simulink model "HPUn_QntBalInjLim"  (R2016b)
settings: configuration reference "CodeGenConfigSet" (kept outside this file)
values from neighbouring files (symbols this model uses):
  HPUn_facPresDvtFlt_C = Calibration.Parameter    [init_HPUn_QntBalInjLim.m]    (also in init_HPUn_QntBalInjLim_SIL.m = Simulink.Parameter)
  HPUn_numInjMin_C = Calibration.Parameter    [init_HPUn_QntBalInjLim.m]    (also in init_HPUn_QntBalInjLim_SIL.m = Simulink.Parameter)
  HPUn_pRailDvtOk_C = Calibration.Parameter    [init_HPUn_QntBalInjLim.m]    (also in init_HPUn_QntBalInjLim_SIL.m = Simulink.Parameter)
  HPUn_tiQntBalDel_C = Calibration.Parameter    [init_HPUn_QntBalInjLim.m]    (also in init_HPUn_QntBalInjLim_SIL.m = Simulink.Parameter)
  InjCrv_numInjMaxSys_C = Calibration.Parameter    [init_HPUn_QntBalInjLim.m]    (also in init_HPUn_QntBalInjLim_SIL.m = Simulink.Parameter)
undefined symbols (not defined in the file or in its folder): HPUn_QntBalInjLim_DT
libraries: CXLib x1
settings Model: Creator=lenovo  LastModifiedBy=lenovo
settings ConfigSetRef: SourceLocation=Base Workspace

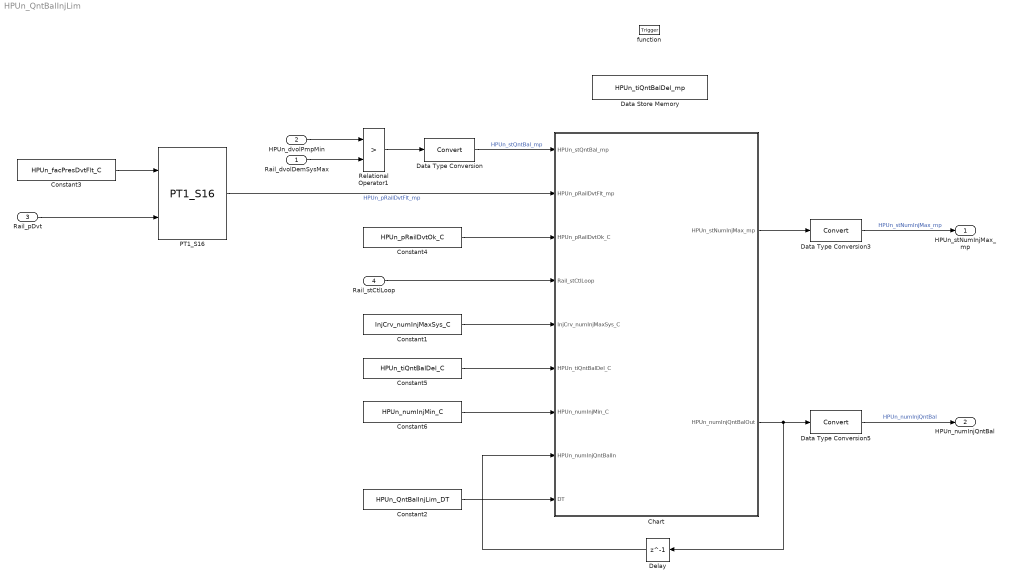
== system HPUn_QntBalInjLim ==
  Rail_dvolDemSysMax : Inport  Tag=mm^3/s  Description=Volume flow requested overall for a maximum tolerated injection system  OutMin=-327680  OutMax=327670  OutDataTypeStr=FuelVol_mm3_s
  HPUn_dvolPmpMin : Inport  Tag=mm^3/s  Description=Minimum pump flow  Port=2  OutMin=0  OutMax=50000  OutDataTypeStr=FuelVol_mm3_s
  Rail_pDvt : Inport  Tag=bar  Description=Governor deviation of the rail pressure governor  Port=3  OutMin=-2500  OutMax=2500  OutDataTypeStr=RailPressure_bar
  Rail_stCtlLoop : Inport  Description=State of the rail pressure governor control  Port=4  OutDataTypeStr=Enum: RailCtl_State_conv
  function : TriggerPort  TriggerType=function-call  VariantControl=Variant
  Chart : Stateflow chart  RequirementInfo={'other' 'HPUn_requirements.docx' '@Simulink_requirement_item_18' 'true' '油量平衡状态判定' '' } %GIDa_78b9b0a6_16aa_4a8d_868e_3e2ef51e585a
  Constant1 : Constant  Value=InjCrv_numInjMaxSys_C
  Constant2 : Constant  Value=HPUn_QntBalInjLim_DT
  Constant3 : Constant  Value=HPUn_facPresDvtFlt_C
  Constant4 : Constant  Value=HPUn_pRailDvtOk_C
  Constant5 : Constant  Value=HPUn_tiQntBalDel_C
  Constant6 : Constant  Value=HPUn_numInjMin_C
  Data Store Memory : DataStoreMemory  DataStoreName=HPUn_tiQntBalDel_mp  ReadBeforeWriteMsg=warning  WriteAfterWriteMsg=warning  WriteAfterReadMsg=warning  ShowAdditionalParam=off  OutDataTypeStr=EngTime_ms  StateMustResolveToSignalObject=on
  Data Type Conversion : DataTypeConversion
  Data Type Conversion3 : DataTypeConversion
  Data Type Conversion5 : DataTypeConversion
  Delay : Delay  DelayLength=1  InitialCondition=0
  PT1_S16 : CXLib/PT1_S16
  Relational Operator1 : RelationalOperator  Operator=>  OutDataTypeStr=boolean  RndMeth=Nearest  InputSameDT=on
  HPUn_stNumInjMax_mp : Outport  Description=Status variable, fuel quantity balance of the high pressure pump  OutMin=0  OutMax=255  OutDataTypeStr=State_uint8
  HPUn_numInjQntBal : Outport  Description=Maximum amount of injections due to high pressure pump quantity balance  Port=2  OutMin=0  OutMax=8  OutDataTypeStr=Counter_num
  wires:
  Constant5/1 -> Chart/6(HPUn_tiQntBalDel_C)
  Chart/1(HPUn_stNumInjMax_mp) -> Data Type Conversion3/1
  Data Type Conversion5/1 -> HPUn_numInjQntBal/1  "HPUn_numInjQntBal"
  Data Type Conversion3/1 -> HPUn_stNumInjMax_mp/1  "HPUn_stNumInjMax_mp"
  PT1_S16/1 -> Chart/2(HPUn_pRailDvtFlt_mp)  "HPUn_pRailDvtFlt_mp"
  Constant3/1 -> PT1_S16/1
  Data Type Conversion/1 -> Chart/1(HPUn_stQntBal_mp)  "HPUn_stQntBal_mp"
  HPUn_dvolPmpMin/1 -> Relational Operator1/1
  Rail_dvolDemSysMax/1 -> Relational Operator1/2
  Relational Operator1/1 -> Data Type Conversion/1
  Delay/1 -> Chart/8(HPUn_numInjQntBalIn)
  Chart/2(HPUn_numInjQntBalOut) -> Delay/1, Data Type Conversion5/1
  Constant6/1 -> Chart/7(HPUn_numInjMin_C)
  Constant1/1 -> Chart/5(InjCrv_numInjMaxSys_C)
  Rail_stCtlLoop/1 -> Chart/4(Rail_stCtlLoop)
  Constant4/1 -> Chart/3(HPUn_pRailDvtOk_C)
  Rail_pDvt/1 -> PT1_S16/2
  Constant2/1 -> Chart/9(DT)

== stateflow chart HPUn_QntBalInjLim/Chart ==
  state QNTBAL_OK
    during:HPUn_stNumInjMax_mp = uint8(0);
    QNTBAL_OK -> (junction 63) [order 1]
    (junction 63) -> (junction 64) [order 1] : [HPUn_tiQntBalDel_mp < HPUn_tiQntBalDel_C]
    (junction 63) -> (junction 65) [order 2] : [HPUn_tiQntBalDel_mp...
        |  >= HPUn_tiQntBalDel_C]
    (junction 64) -> (junction 69) : {HPUn_tiQntBalDel_mp = HPUn_tiQntBalDel_mp + DT;}
    (junction 65) -> (junction 66) [order 1] : [HPUn_numInjQntBalIn...
        |  < InjCrv_numInjMaxSys_C]
    (junction 65) -> (junction 67) [order 2] : {HPUn_numInjQntBalOut = InjCrv_numInjMaxSys_C;}
    (junction 66) -> (junction 68) : {HPUn_numInjQntBalOut = HPUn_numInjQntBalIn + 1;}
    (junction 68) -> (junction 67)
    (junction 69) -> (junction 68)
    (junction 67) -> (junction 70)
  state QNTBAL_NOT_OK
    during:HPUn_stNumInjMax_mp = uint8(1);
    QNTBAL_NOT_OK -> (junction 86) [order 1]
    (junction 86) -> (junction 87) [order 1] : [HPUn_tiQntBalDel_mp < HPUn_tiQntBalDel_C]
    (junction 86) -> (junction 88) [order 2] : [HPUn_tiQntBalDel_mp...
        |  >= HPUn_tiQntBalDel_C]
    (junction 87) -> (junction 92) : {HPUn_tiQntBalDel_mp = HPUn_tiQntBalDel_mp + DT;}
    (junction 88) -> (junction 89) [order 1] : [HPUn_numInjQntBalIn...
        |  > HPUn_numInjMin_C]
    (junction 88) -> (junction 90) [order 2] : {HPUn_numInjQntBalOut = HPUn_numInjMin_C;}
    (junction 89) -> (junction 91) : {HPUn_numInjQntBalOut = HPUn_numInjQntBalIn - 1;}
    (junction 91) -> (junction 90)
    (junction 92) -> (junction 91)
    (junction 90) -> (junction 93)
  (default) -> QNTBAL_OK
  QNTBAL_OK -> QNTBAL_NOT_OK [order 1] : [(HPUn_stQntBal_mp == 0)&&...
      | (HPUn_pRailDvtFlt_mp > HPUn_pRailDvtOk_C) &&...
      | ((Rail_stCtlLoop == RailCtl_State_conv.RAIL_CTL_PCV)||...
      | (Rail_stCtlLoop == RailCtl_State_conv.RAIL_CTL_MEUN)||...
      | (Rail_stCtlLoop == RailCtl_State_conv.RAIL_CTL_CPC)|| ...
      | (Rail_stCtlLoop == RailCtl_State_conv.RAIL_SWT_PRECTL_PCV )||...
      | (Rail_stCtlLoop == RailCtl_State_conv.RAIL_SWT_CTL_CPC)||...
      | (Rail_stCtlLoop == RailCtl_State_conv.RAIL_SWT_PRECTL_MEUN))]
      | {HPUn_tiQntBalDel_mp = 0;}
  QNTBAL_NOT_OK -> QNTBAL_OK [order 1] : [(HPUn_stQntBal_mp == 1)||...
      | ((Rail_stCtlLoop ~= RailCtl_State_conv.RAIL_CTL_PCV)&&...
      | (Rail_stCtlLoop ~= RailCtl_State_conv.RAIL_CTL_MEUN)&&...
      | (Rail_stCtlLoop ~= RailCtl_State_conv.RAIL_CTL_CPC)&&...
      | (Rail_stCtlLoop ~= RailCtl_State_conv.RAIL_SWT_PRECTL_PCV)&&...
      | (Rail_stCtlLoop ~= RailCtl_State_conv.RAIL_SWT_CTL_CPC)&&...
      | (Rail_stCtlLoop ~= RailCtl_State_conv.RAIL_SWT_PRECTL_MEUN))]
      | {HPUn_tiQntBalDel_mp = 0;}
  data: HPUn_stNumInjMax_mp output uint8; HPUn_stQntBal_mp input; HPUn_pRailDvtFlt_mp input; HPUn_pRailDvtOk_C input; Rail_stCtlLoop input; HPUn_numInjQntBalOut output uint16; InjCrv_numInjMaxSys_C input; HPUn_tiQntBalDel_C input; HPUn_numInjMin_C input; HPUn_numInjQntBalIn input; HPUn_tiQntBalDel_mp data_store_memory =0; DT input
